simulink model "homework602"  (R2019b)
settings: Solver=VariableStepAuto  StartTime=0.0  StopTime=50  RelTol=1e-3
libraries: simulink_extras x4
settings Model: Creator=路西法  LastModifiedBy=Lenovo
settings DataIOCC: ReturnWorkspaceOutputs=off
settings DebuggingCC: ArithmeticOperatorsInVariantConditions=warning
settings SFSimCC: SimUseLocalCustomCode=off  CustomCodeUndefinedFunction=UseInterfaceOnly
settings RTWCC: RTWUseLocalCustomCode=off

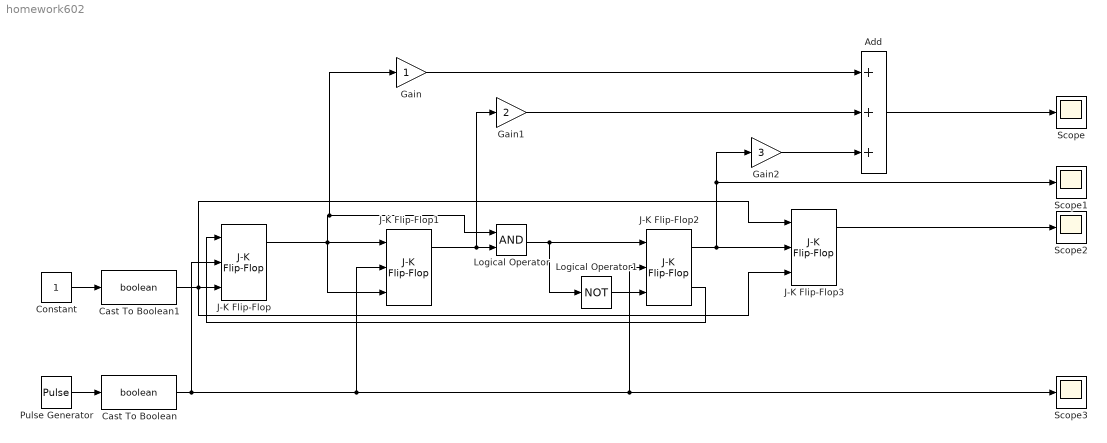
== system homework602 ==
  Add : Sum  Inputs=3
  Cast To Boolean : DataTypeConversion  OutDataTypeStr=boolean
  Cast To Boolean1 : DataTypeConversion  OutDataTypeStr=boolean
  Constant : Constant
  Gain : Gain
  Gain1 : Gain  Gain=2
  Gain2 : Gain  Gain=3
  J-K Flip-Flop{,1..3} (4 alike) : simulink_extras/Flip Flops/J-K Flip-Flop  initial_condition=0
      settings: SourceProductName=Simulink
  Logical Operator : Logic  AllPortsSameDT=off  OutDataTypeStr=boolean
  Logical Operator1 : Logic  Operator=NOT  AllPortsSameDT=off  OutDataTypeStr=boolean
  Pulse Generator : DiscretePulseGenerator  PhaseDelay=1
  Scope{,1..3} (4 alike) : Scope
  wires:
  J-K Flip-Flop/1 -> J-K Flip-Flop1/3, Gain/1, Logical Operator/1, J-K Flip-Flop1/1
  J-K Flip-Flop1/1 -> Gain1/1, Logical Operator/2
  Logical Operator/1 -> Logical Operator1/1, J-K Flip-Flop2/1
  Logical Operator1/1 -> J-K Flip-Flop2/3
  J-K Flip-Flop2/2 -> J-K Flip-Flop/1
  Constant/1 -> Cast To Boolean1/1
  Pulse Generator/1 -> Cast To Boolean/1
  Cast To Boolean/1 -> Scope3/1, J-K Flip-Flop2/2, J-K Flip-Flop1/2, J-K Flip-Flop/2
  J-K Flip-Flop2/1 -> Scope1/1, Gain2/1, J-K Flip-Flop3/2
  Cast To Boolean1/1 -> J-K Flip-Flop3/1, J-K Flip-Flop3/3, J-K Flip-Flop/3
  Gain/1 -> Add/1
  Gain1/1 -> Add/2
  Gain2/1 -> Add/3
  Add/1 -> Scope/1
  J-K Flip-Flop3/1 -> Scope2/1
